simulink model "mrac_paper_no_disturbance"  (R2018a)
settings: Solver=VariableStepAuto  StartTime=0.0  StopTime=120.0  MaxStep=1e-2  RelTol=1e-3
settings Model: Creator=saad  LastModifiedBy=saad

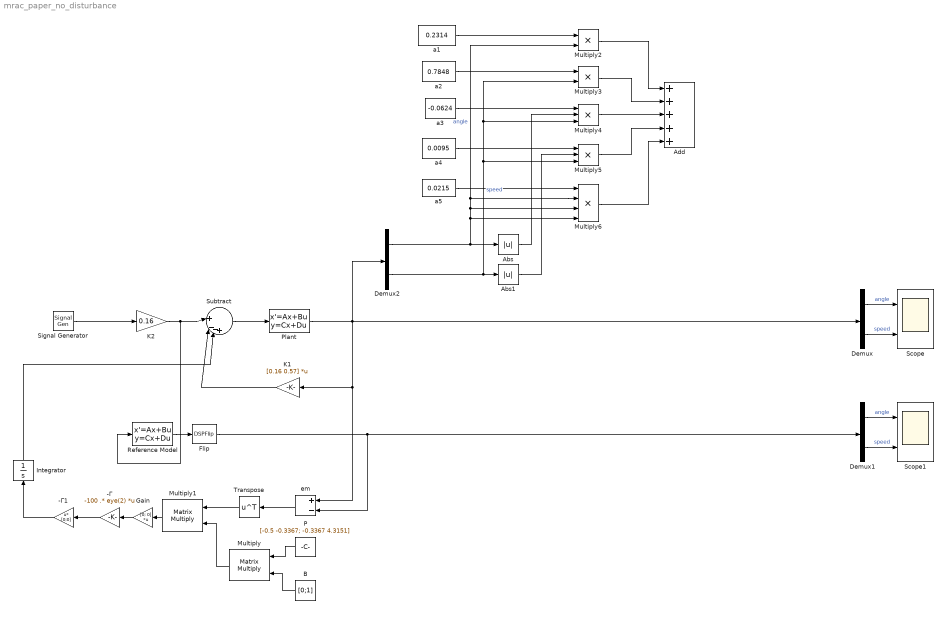
== system mrac_paper_no_disturbance ==
  -Γ : Gain  Gain=-100 .* eye(2)  Multiplication=Matrix(K*u)
  -Γ1 : Gain  Gain=[0;0]  Multiplication=Matrix(u*K)
  Abs : Abs
  Abs1 : Abs
  Add : Sum  Inputs=+++++
  B : Constant  Value=[0;1]
  Demux : Demux  Outputs=2
  Demux1 : Demux  Outputs=2
  Demux2 : Demux  Outputs=2
  Flip : DSPFlip
  Gain : Gain  Gain=[0; 0]  Multiplication=Matrix(K*u)
  Integrator : Integrator
  K1 : Gain  Gain=[0.16 0.57]  Multiplication=Matrix(K*u)
  K2 : Gain  Gain=0.16
  Multiply : Product  Multiplication=Matrix(*)
  Multiply1 : Product  Multiplication=Matrix(*)
  Multiply2 : Product
  Multiply3 : Product
  Multiply4 : Product  Inputs=3
  Multiply5 : Product  Inputs=3
  Multiply6 : Product  Inputs=4
  P : Constant  Value=[-0.5 -0.3367; -0.3367 4.3151]
  Plant : StateSpace  A=[0 1;0 0]  B=[0;1]  C=eye(2)  D=[0;0]  InitialCondition=0  ContinuousStateAttributes={'x1', 'x2'}
  Reference Model : StateSpace  A=[-0.5656, -0.16; 1,0]  B=[1;0]  C=eye(2)  D=[0;0]  InitialCondition=0
  Scope : Scope  NumInputPorts=2
  Scope1 : Scope  NumInputPorts=2
  Signal Generator : SignalGenerator  WaveForm=square  Amplitude=-15  Frequency=pi/30  Units=rad/sec
  Subtract : Sum  Inputs=|||+|--+
  Transpose : Math  Operator=transpose  SaturateOnIntegerOverflow=on
  a1 : Constant  Value=0.2314
  a2 : Constant  Value=0.7848
  a3 : Constant  Value=-0.0624
  a4 : Constant  Value=0.0095
  a5 : Constant  Value=0.0215
  em : Sum  Inputs=+-
  wires:
  Signal Generator/1 -> K2/1
  K2/1 -> Reference Model/1, Subtract/1
  K1/1 -> Subtract/2
  Subtract/1 -> Plant/1
  Demux/1 -> Scope/1  "angle"
  Demux/2 -> Scope/2  "speed"
  Demux1/1 -> Scope1/1  "angle"
  Demux1/2 -> Scope1/2  "speed"
  Reference Model/1 -> Flip/1
  Flip/1 -> em/2, Demux1/1
  P/1 -> Multiply/1
  B/1 -> Multiply/2
  Multiply/1 -> Multiply1/2
  em/1 -> Transpose/1
  Transpose/1 -> Multiply1/1
  Gain/1 -> -Γ/1
  Multiply1/1 -> Gain/1
  -Γ/1 -> -Γ1/1
  -Γ1/1 -> Integrator/1
  Demux2/1 -> Abs/1, Multiply6/4, Multiply6/3, Multiply6/2, Multiply2/2  "angle"
  Demux2/2 -> Abs1/1, Multiply5/3, Multiply4/3, Multiply3/2  "speed"
  Plant/1 -> Demux/1, Demux2/1, em/1, K1/1
  a1/1 -> Multiply2/1
  a2/1 -> Multiply3/1
  a3/1 -> Multiply4/1
  a4/1 -> Multiply5/1
  a5/1 -> Multiply6/1
  Abs/1 -> Multiply4/2
  Abs1/1 -> Multiply5/2
  Multiply4/1 -> Add/3
  Multiply3/1 -> Add/2
  Multiply2/1 -> Add/1
  Multiply5/1 -> Add/4
  Multiply6/1 -> Add/5
  Integrator/1 -> Subtract/3
